simulink model "P1_Seniales_y_Sistemas"  (R2020a)
settings: Solver=VariableStepAuto  StartTime=0.0  StopTime=1  RelTol=1e-3
libraries: commchan3 x1
settings Model: Creator=León Mora  LastModifiedBy=León Mora

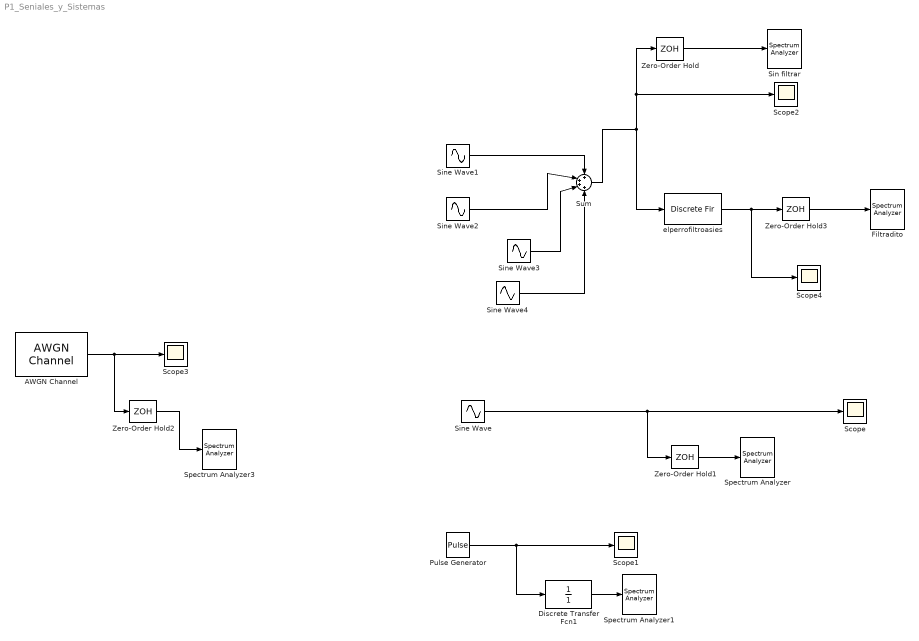
== system P1_Seniales_y_Sistemas ==
  AWGN Channel : commchan3/AWGN Channel  InputProcessing=Columns as channels (frame based)  seed=67  noiseMode=Variance from mask  EbNodB=10  EsNodB=10  SNRdB=10  bitsPerSym=1  Ps=1  Tsym=1  variance=0.1
  Discrete Transfer Fcn1 : DiscreteTransferFcn  Numerator=1  Denominator=1  SampleTime=1/5000
  Filtradito : SpectrumAnalyzer
  Pulse Generator : DiscretePulseGenerator  PulseType=Time based  Period=0.1  PulseWidth=25
  Scope{,1..4} (5 alike) : Scope
  Sin filtrar : SpectrumAnalyzer
  Sine Wave : Sin  Amplitude=5  Frequency=2400*pi  SampleTime=0
  Sine Wave1 : Sin  Frequency=2000*2*pi  SampleTime=0
  Sine Wave2 : Sin  Frequency=4000*2*pi  SampleTime=0
  Sine Wave3 : Sin  Frequency=8000*2*pi  SampleTime=0
  Sine Wave4 : Sin  Frequency=10000*2*pi  SampleTime=0
  Spectrum Analyzer : SpectrumAnalyzer
  Spectrum Analyzer1 : SpectrumAnalyzer
  Spectrum Analyzer3 : SpectrumAnalyzer
  Sum : Sum  Inputs=++++
  Zero-Order Hold{,1..3} (4 alike) : ZeroOrderHold  SampleTime=1e-5
  elperrofiltroasies : DiscreteFir  Tag=BlockMethodSubSystem  Coefficients=[0.146267295807684578 0.707465408384630789 0.146267295807684578]  InputProcessing=Columns as channels (frame based)  SampleTime=1e-5
  wires:
  Sine Wave/1 -> Zero-Order Hold1/1, Scope/1
  Pulse Generator/1 -> Scope1/1, Discrete Transfer Fcn1/1
  Sine Wave3/1 -> Sum/3
  Sine Wave4/1 -> Sum/4
  Sine Wave1/1 -> Sum/1
  Sine Wave2/1 -> Sum/2
  Sum/1 -> elperrofiltroasies/1, Zero-Order Hold/1, Scope2/1
  AWGN Channel/1 -> Zero-Order Hold2/1, Scope3/1
  Zero-Order Hold/1 -> Sin filtrar/1
  Zero-Order Hold1/1 -> Spectrum Analyzer/1
  Discrete Transfer Fcn1/1 -> Spectrum Analyzer1/1
  Zero-Order Hold2/1 -> Spectrum Analyzer3/1
  elperrofiltroasies/1 -> Zero-Order Hold3/1, Scope4/1
  Zero-Order Hold3/1 -> Filtradito/1
